simulink model "VDCHyd2022a"  (R2022a)
settings: Solver=daessc  StartTime=0.0  StopTime=simulationEndTime  FixedStep=0.001  RelTol=1e-2
values from neighbouring files (symbols this model uses):
  aux = thetaXrLB(i)    [initInertiaUpdate.m]
  Bc1_V = [0;0;0;0;0;0]    [InitializeSimulationParameters.m]
  Bc1_Vr = [0;0;0;0;0;0]    [InitializeSimulationParameters.m]
  D22Fr = [0;0;0;0;0;0]    [InitializeSimulationParameters.m]
  filtDF = init2ndOrderLowPassFilter(filtDF.cutOffFrequency,1,controller.dT)    [initializeLowPassFilters.m]
  filtDV = init2ndOrderLowPassFilter(filtDV.cutOffFrequency,1,controller.dT)    [initializeLowPassFilters.m]
  filtEnc = init2ndOrderLowPassFilter(filtEnc.cutOffFrequency,1,controller.dT)    [initializeLowPassFilters.m]
  filtPres = init2ndOrderLowPassFilter(filtPres.cutOffFrequency,1,controller.dT)    [initializeLowPassFilters.m]
  MODE = 1    [RUN_ME.m]
  s = tf('s')    [init2ndOrderLowPassFilter.m]
undefined symbols (not defined in the file or in its folder): B11_r_B11Tc1, B11_V, B11_Vr, B11Ftot_r, B12_r_B12Tc2, B12_Rot_Tc2, B12_U_Tc2, B12_V, B12_Vr, B12Ftot_r, B31_r_B31B41, B31_V, B31_Vr, B31FTot_r, B32_r_B32B42, B32_Rot_B42, B32_U_B42, B32_V, B32_Vr, B32FTot_r, B41_r_B41Tc1, B41_V, B41_Vr, B41FTot_r, B42_r_B42Tc2, B42_Rot_Tc2, B42_U_Tc2, B42_V, B42_Vr, B42FTot_r, B52_r_B52P32, B52_Rot_P32, B52_U_P32, B52_V, B52_Vr, B52Ftot_r, Bc1_r_Bc1B11, Bc1_r_Bc1B31, Bc1FTot_r, Bc2_r_Bc2B12, Bc2_r_Bc2B32, Bc2_Rot_B12, Bc2_Rot_B32, Bc2_U_B12, Bc2_U_B32, Bc2_V, Bc2_Vr, Bc2Tot_r, controller, cyl1, cyl2, cylT2, D22_V, D22_Vr, DiscIntNeverNeededParam, dq1, dq11, dq11r, dq12, dq12r ... (+119)
libraries: sm_lib x34, nesl_utility x15, simulink x11, dspinverses x1
(part 1 of 12)
settings Model: SimulationMode=accelerator  Creator=liikaneh  LastModifiedBy=pvgope
settings SolverCC: AlgebraicLoopSolver=TrustRegion
settings OptimizationCC: DefaultParameterBehavior=Inlined  GainParamInheritBuiltInType=on  UseFloatMulNetSlope=on  InlineInvariantSignals=on  EfficientFloat2IntCast=on
settings DebuggingCC: ReadBeforeWriteMsg=DisableAll  WriteAfterWriteMsg=DisableAll  WriteAfterReadMsg=DisableAll  MultiTaskDSMMsg=none  UnconnectedInputMsg=warning  UnconnectedOutputMsg=warning  UnconnectedLineMsg=warning  SFMachineParentedDataDiag=warning  ArithmeticOperatorsInVariantConditions=warning
settings ModelReferenceCC: UpdateModelReferenceTargets=IfOutOfDate
settings SFSimCC: SFSimEcho=off  SimUseLocalCustomCode=off  CustomCodeUndefinedFunction=UseInterfaceOnly
settings RTWCC: RTWUseLocalCustomCode=off  BuildConfiguration=Faster Runs  DLArmComputeVersion=19.05
settings GRTTargetCC: MatFileLogging=off  SupportNonFinite=off
settings DiagnosticsConfigSet: SimMechanicsRigidlyBoundBlock=none

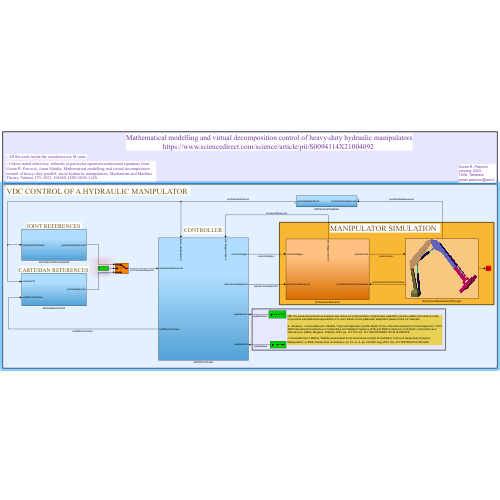
[thumbnail: Simulink's stored preview of the top-level diagram]
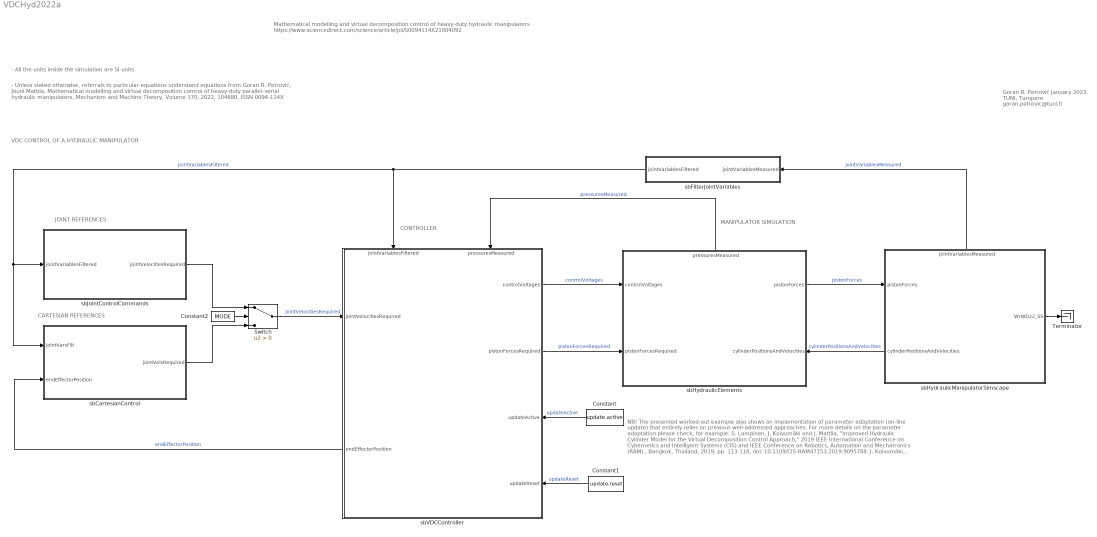
== system VDCHyd2022a ==
  note: NB! The presented worked-out example also shows an implementation of parameter adaptation (on-line update) that entirely relies on previous well-addressed approaches. For more details on the parameter adaptation please check, for example:
      |
      | S. Lampinen, J. Koivumäki and J. Mattila, "Improved Hydraulic Cylinder Model for the Virtual Decomposition Control Approach," 2019 IEEE International Conference on Cybernetics and Intelligent Systems (CIS) and IEEE Conference on Robotics, Automation and Mechatronics (RAM) , Bangkok, Thailand, 2019, pp. 113-118, doi: 10.1109/CIS-RAM47153.2019.9095788.
      |
      | J. Koivumäki and J. Mattila, "Stability-Guaranteed Force-Sensorless Contact Force/Motion Control of Heavy-Duty Hydraulic Manipulators," in IEEE Transactions on Robotics , vol. 31, no. 4, pp. 918-935, Aug. 2015, doi: 10.1109/TRO.2015.2441492.
  note: Mathematical modelling and virtual decomposition control of heavy-duty hydraulic manipulators
      | https://www.sciencedirect.com/science/article/pii/S0094114X21004092
  note: Goran R. Petrović
      | January 2023.
      | TUNI, Tampere
      | goran.petrovic@tuni.fi
  note: - All the units inside the simulation are SI units.
  note: - Unless stated otherwise, referrals to particular equations understand equations from Goran R. Petrović, Jouni Mattila, Mathematical modelling and virtual decomposition control of heavy-duty parallel–serial hydraulic manipulators, Mechanism and Machine Theory, Volume 170, 2022, 104680, ISSN 0094-114X
  note: MANIPULATOR SIMULATION
  note: VDC CONTROL OF A HYDRAULIC MANIPULATOR
  note: JOINT REFERENCES
  note: CARTESIAN REFERENCES
  note: CONTROLLER
  Constant : Constant  Value=update.active
  Constant1 : Constant  Value=update.reset
  Constant2 : Constant  Value=MODE
  Switch : Switch  Criteria=u2 > Threshold  SaturateOnIntegerOverflow=off  InputSameDT=off
  Terminator : Terminator
  sbCartesianControl : Subsystem
  sbFilterJointVariables : Subsystem
  sbHydraulicElements : Subsystem
      settings: PortSchema="{\"entries\":[{\"content\":{\"sides\":[{\"content\":{\"connectorIds\":[\"In1\",\"In2\"]},\"type\":\"ConnectorPlacement.EquallySpacedRectSide\",\"uuid\":\"d7e88d44-ea3b-4e6f-b434-d63e26d49c99\"},{\"content\":{\"connectorIds\":[\"Out1\",\"In3\"],\"side\":\"RIGHT\"},\"type\":\"ConnectorPlacement.EquallySpacedRectSide\",\"uuid\":\"625eb6db-a413-4233-8471-3960265b5680\"},{\"content\":{\"connectorIds\":[\"Out2\"],\"side\":\"TOP\"},\"type\":\"ConnectorPlacement.EquallySpacedRectSide\",\"uuid\":\"1363109f-1b18-4a4e-ba16-4e74caafe6c6\"}]},\"type\":\"ConnectorPlacement.EquallySpacedConnector\",\"uuid\":\"f039fec2-5503-4fd9-bf11-cf75dff43144\"}],\"packageUris\":[\"http://schema.mathworks.com/mf0/Connector/R2020b\"],\"version\":\"1.0\"}"
  sbHydraulicManipulatorSimscape : Subsystem
      settings: PortSchema="{\"entries\":[{\"content\":{\"sides\":[{\"content\":{\"connectorIds\":[\"In1\",\"Out3\"]},\"type\":\"ConnectorPlacement.EquallySpacedRectSide\",\"uuid\":\"f7b00952-2d51-484f-abea-a7edf7f1803a\"},{\"content\":{\"connectorIds\":[\"Out1\"],\"side\":\"RIGHT\"},\"type\":\"ConnectorPlacement.EquallySpacedRectSide\",\"uuid\":\"cec57a8d-f407-43fc-b54f-695abbd67ebc\"},{\"content\":{\"connectorIds\":[\"Out2\"],\"side\":\"TOP\"},\"type\":\"ConnectorPlacement.EquallySpacedRectSide\",\"uuid\":\"36c8b0b2-f27a-4d8c-8e2c-18a80d711d3e\"}]},\"type\":\"ConnectorPlacement.EquallySpacedConnector\",\"uuid\":\"9ce8286e-5e91-4ec7-b364-968722180a48\"}],\"packageUris\":[\"http://schema.mathworks.com/mf0/Connector/R2020b\"],\"version\":\"1.0\"}"
      mask Display: image('$imagefile'); % Use "Edit Image" on toolstrip to change.
  sbJointControlCommands : Subsystem
  sbVDCController : Subsystem
      settings: PortSchema="{\"entries\":[{\"content\":{\"sides\":[{\"content\":{\"connectorIds\":[\"In1\",\"Out3\"]},\"type\":\"ConnectorPlacement.EquallySpacedRectSide\",\"uuid\":\"7b05da7d-8e98-4260-b965-883aeff80f6d\"},{\"content\":{\"connectorIds\":[\"Out1\",\"Out2\",\"In4\",\"In5\"],\"side\":\"RIGHT\"},\"type\":\"ConnectorPlacement.EquallySpacedRectSide\",\"uuid\":\"bab503f6-0cf2-4d25-8612-166524dadf44\"},{\"content\":{\"connectorIds\":[\"In2\",\"In3\"],\"side\":\"TOP\"},\"type\":\"ConnectorPlacement.EquallySpacedRectSide\",\"uuid\":\"dc9bf139-dfcc-4316-b9ab-c299ea19db13\"}]},\"type\":\"ConnectorPlacement.EquallySpacedConnector\",\"uuid\":\"a723f5e0-c36b-4f3a-b452-df4ada5825ab\"}],\"packageUris\":[\"http://schema.mathworks.com/mf0/Connector/R2020b\"],\"version\":\"1.0\"}"
  wires:
  sbVDCController/1(controlVoltages) -> sbHydraulicElements/1(controlVoltages)  "controlVoltages"
  sbHydraulicElements/1(pistonForces) -> sbHydraulicManipulatorSimscape/1(pistonForces)  "pistonForces"
  Switch/1 -> sbVDCController/1(jointVelocitiesRequired)  "jointVelocitiesRequired"
  sbHydraulicManipulatorSimscape/2(jointVariablesMeasured) -> sbFilterJointVariables/1(jointVariablesMeasured)  "jointVariablesMeasured"
  sbFilterJointVariables/1(jointVariablesFiltered) -> sbVDCController/2(jointVariablesFiltered), sbCartesianControl/1(jointVarsFilt), sbJointControlCommands/1(jointVariablesFiltered)  "jointVariablesFiltered"
  sbHydraulicManipulatorSimscape/1(WrWD22_SS) -> Terminator/1
  sbVDCController/2(pistonForcesRequired) -> sbHydraulicElements/2(pistonForcesRequired)  "pistonForcesRequired"
  sbHydraulicElements/2(pressuresMeasured) -> sbVDCController/3(pressuresMeasured)  "pressuresMeasured"
  Constant/1 -> sbVDCController/4(updateActive)  "updateActive"
  Constant1/1 -> sbVDCController/5(updateReset)  "updateReset"
  sbVDCController/3(endEffectorPosition) -> sbCartesianControl/2(endEffectorPosition)  "endEffectorPosition"
  sbHydraulicManipulatorSimscape/3(cylinderPositionsAndVelocities) -> sbHydraulicElements/3(cylinderPositionsAndVelocities)  "cylinderPositionsAndVelocities"
  sbJointControlCommands/1(jointVelocitiesRequired) -> Switch/1
  sbCartesianControl/1(jointVelsRequired) -> Switch/3
  Constant2/1 -> Switch/2

== system VDCHyd2022a/sbCartesianControl ==
  note: Pass to outputs...
  note: Process data...
  note: Select from existing buses...
  note: X^{'}_r = X^{'}_d + \lambda_X (X - X_d)
  note: (3.22) W. H. Zhu, Virtual decomposition control: toward hyper degrees of freedom robots, pp. 51
  note: (3.21) W. H. Zhu, Virtual decomposition control: toward hyper degrees of freedom robots, pp. 51
  note: (3.21) W. H. Zhu, Virtual decomposition control: toward hyper degrees of freedom robots, pp. 51
  note: Get inputs...
  note: Y^{'}_r = Y^{'}_d + \lambda_Y (Y - Y_d)
  note: q^{'}_r = J^{ -1} V^{'}_r
  note: Compare desired and obtained TCP positions.
  jointVarsFilt : Inport
  endEffectorPosition : Inport  Port=2
  Bus Selector : BusSelector  OutputSignals=theta1Filtered,theta2Filtered,xt2Filtered
  Demux2 : Demux  Outputs=3
  From Workspace : FromWorkspace  VariableName=[pathPlanner.timeVector' pathPlanner.posDesCart(1,1:end)']  SampleTime=controller.dT
  From Workspace1 : FromWorkspace  VariableName=[pathPlanner.timeVector' pathPlanner.posDesCart(2,1:end)']  SampleTime=controller.dT
  From Workspace2 : FromWorkspace  VariableName=[pathPlanner.timeVector' pathPlanner.velDesCart(1,1:end)']  SampleTime=controller.dT
  From Workspace3 : FromWorkspace  VariableName=[pathPlanner.timeVector' pathPlanner.velDesCart(2,1:end)']  SampleTime=controller.dT
  Gain : Gain  Gain=controller.lamX
  Gain1 : Gain  Gain=controller.lamY
  Mux1 : Mux  Inputs=2
  Product : Product  Multiplication=Matrix(*)
  Pseudoinverse : dspinverses/Pseudoinverse  wanterr=off  SimulateUsing=Interpreted execution
      settings: SourceProductBaseCode=DS
  Scope : Scope  NumInputPorts=2
  Scope1 : Scope  NumInputPorts=2
  Sum3 : Sum  Inputs=|+-
  Sum4 : Sum  Inputs=|+-
  Sum5 : Sum  Inputs=|++
  Sum6 : Sum  Inputs=|++
  Terminator1 : Terminator
  velocityJacobianFunction : MATLAB Function  TreatAsAtomicUnit=on
  jointVelsRequired : Outport
  wires:
  [xt2Filt] -> velocityJacobianFunction/3(xt2)  "xt2Filt"
  [theta2Filt] -> velocityJacobianFunction/2(theta2)  "theta2Filt"
  Product/1 -> [jointVelsRequired]
  Mux1/1 -> Product/2
  velocityJacobianFunction/1(J) -> Pseudoinverse/1
  [theta1Filt] -> velocityJacobianFunction/1(theta1)  "theta1Filt"
  Pseudoinverse/1 -> Product/1
  [jointVelsRequired] -> jointVelsRequired/1  "jointVelsRequired"
  [XVelReq] -> Mux1/1
  [YVelReq] -> Mux1/2
  [XDes] -> Sum3/1
  [X] -> Sum3/2
  [YDes] -> Sum4/1
  [Y] -> Sum4/2
  Sum3/1 -> Gain/1
  Sum4/1 -> Gain1/1
  Gain/1 -> Sum5/1
  Gain1/1 -> Sum6/1
  [XVelDes] -> Sum5/2
  [YVelDes] -> Sum6/2
  Sum5/1 -> [XVelReq]
  Sum6/1 -> [YVelReq]
  [X] -> Scope/2
  [XDes] -> Scope/1
  [YDes] -> Scope1/1
  [Y] -> Scope1/2
  From Workspace/1 -> [XDes]
  From Workspace1/1 -> [YDes]
  From Workspace3/1 -> [YVelDes]
  From Workspace2/1 -> [XVelDes]
  [jointVarsFilt] -> Bus Selector/1  "jointVarsFilt"
  Bus Selector/3 -> [xt2Filt]  "<xt2Filtered>"
  Bus Selector/2 -> [theta2Filt]  "<theta2Filtered>"
  Bus Selector/1 -> [theta1Filt]  "<theta1Filtered>"
  Demux2/1 -> [X]  "X"
  Demux2/2 -> [Y]  "Y"
  Demux2/3 -> Terminator1/1
  [endEffectorPosition] -> Demux2/1  "WrWD22"
  jointVarsFilt/1 -> [jointVarsFilt]  "jointVarsFilt"
  endEffectorPosition/1 -> [endEffectorPosition]  "WrWD22"

== system VDCHyd2022a/sbFilterJointVariables ==
  jointVariablesMeasured : Inport  OutDataTypeStr=double  PortDimensions=3  SampleTime=controller.dT
  Bus Creator : BusCreator  Inputs=theta1Filtered,theta2Filtered,xt2Filtered
  Bus Selector : BusSelector  OutputSignals=theta1Measured,theta2Measured,xt2Measured
  sbTheta1LowPassFilter : Subsystem
  sbTheta2LowPassFilter : Subsystem
  sbxt2LowPassFilter : Subsystem
  jointVariablesFiltered : Outport  OutDataTypeStr=double  PortDimensions=3  SampleTime=controller.dT
  wires:
  sbxt2LowPassFilter/1(xt2Filtered) -> Bus Creator/3  "xt2Filtered"
  sbTheta2LowPassFilter/1(theta2Filtered) -> Bus Creator/2  "theta2Filtered"
  sbTheta1LowPassFilter/1(theta1Filtered) -> Bus Creator/1  "theta1Filtered"
  Bus Selector/2 -> sbTheta2LowPassFilter/1(theta2Measured)  "<theta2Measured>"
  Bus Selector/1 -> sbTheta1LowPassFilter/1(theta1Measured)  "<theta1Measured>"
  Bus Selector/3 -> sbxt2LowPassFilter/1(xt2Measured)  "<xt2Measured>"
  jointVariablesMeasured/1 -> Bus Selector/1  "jointVariablesMeasured"
  Bus Creator/1 -> jointVariablesFiltered/1  "jointVariablesFiltered"

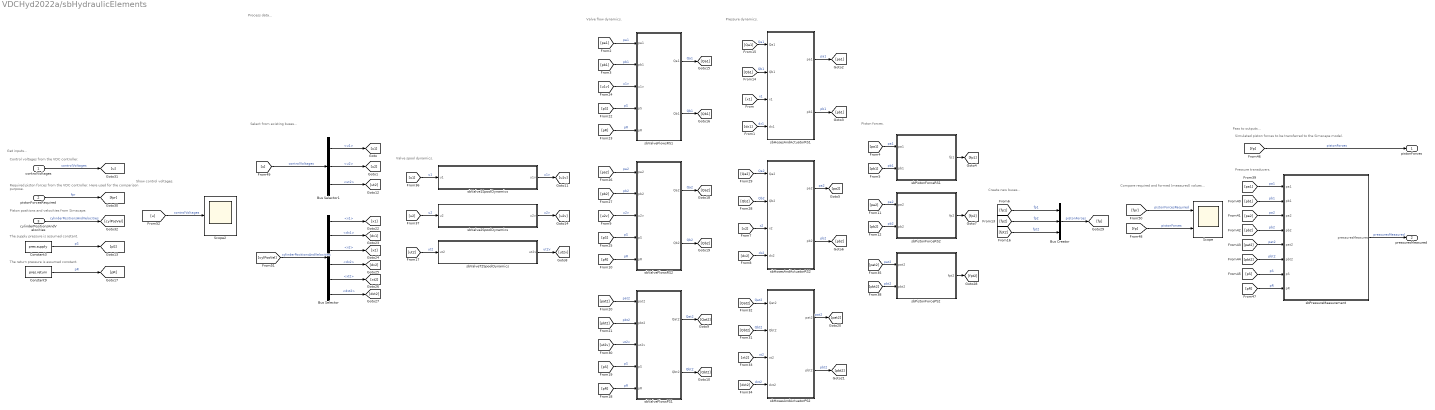
== system VDCHyd2022a/sbHydraulicElements ==
  note: Pass to outputs...
  note: Process data...
  note: Simulated piston forces to be transferred to the Simscape model.
  note: Pressure transducers.
  note: Create new buses...
  note: Select from existing buses...
  note: Piston positions and velocities from Simscape.
  note: Control voltages from the VDC controller.
  note: Required piston forces from the VDC controller.
      | Here used for the comparison purpose.
  note: Get inputs...
  note: The supply pressure is assumed constant.
  note: Valve spool dynamics.
  note: The return pressure is assumed constant.
  note: Piston forces.
  note: Pressure dynamics.
  note: Valve flow dynamics.
  note: Compare required and formed (measured) values...
  note: Show control voltages.
  controlVoltages : Inport
  pistonForcesRequired : Inport  Port=2
  cylinderPositionsAndVelocities : Inport  Port=3
  Bus Creator : BusCreator  Inputs=fp1,fp2,fpt2
  Bus Selector : BusSelector  OutputSignals=x1,dx1,x2,dx2,xt2,dxt2
  Bus Selector1 : BusSelector  OutputSignals=u1,u2,ut2
  Constant3 : Constant  Value=pres.supply
  Constant9 : Constant  Value=pres.return
  Scope : Scope  NumInputPorts=2
  Scope2 : Scope
  sbHosesAndActuatorPS2 : Subsystem
  sbHosesAndActuatorRS1 : Subsystem
  sbHosesAndActuatorRS2 : Subsystem
  sbPistonForcePS2 : Subsystem
  sbPistonForceRS1 : Subsystem
  sbPistonForceRS2 : Subsystem
  sbPressureMeasurement : Subsystem
  sbValve1SpoolDynamics : Subsystem
  sbValve2SpoolDynamics : Subsystem
  sbValveFlowsPS1 : Subsystem
  sbValveFlowsRS1 : Subsystem
  sbValveFlowsRS2 : Subsystem
  sbValveT2SpoolDynamics : Subsystem
  pistonForces : Outport
  pressuresMeasured : Outport  Port=2
  wires:
  [u1v] -> sbValveFlowsRS1/3(u1v)  "u1v"
  [Qb2] -> sbHosesAndActuatorRS2/2(Qb2)  "Qb2"
  sbValveFlowsRS2/1(Qa2) -> [Qa2]  "Qa2"
  [u2] -> sbValve2SpoolDynamics/1(u2)  "u2"
  [pS] -> sbValveFlowsRS1/4(pS)  "pS"
  [u2v] -> sbValveFlowsRS2/3(u2v)  "u2v"
  sbValveFlowsRS2/2(Qb2) -> [Qb2]  "Qb2"
  [dx2] -> sbHosesAndActuatorRS2/4(dx2)  "dx2"
  [pa2] -> sbValveFlowsRS2/1(pa2)  "pa2"
  [pb1] -> sbValveFlowsRS1/2(pb1)  "pb1"
  [dx1] -> sbHosesAndActuatorRS1/4(dx1)  "dx1"
  sbValveFlowsRS1/1(Qa1) -> [Qa1]  "Qa1"
  [pa1] -> sbValveFlowsRS1/1(pa1)  "pa1"
  [pR] -> sbValveFlowsRS1/5(pR)  "pR"
  sbHosesAndActuatorRS2/2(pb2) -> [pb2]  "pb2"
  [Qa2] -> sbHosesAndActuatorRS2/1(Qa2)  "Qa2"
  [Qa1] -> sbHosesAndActuatorRS1/1(Qa1)  "Qa1"
  Constant9/1 -> [pR]  "pR"
  [Qb1] -> sbHosesAndActuatorRS1/2(Qb1)  "Qb1"
  [pb2] -> sbValveFlowsRS2/2(pb2)  "pb2"
  sbHosesAndActuatorRS1/1(pa1) -> [pa1]  "pa1"
  [x2] -> sbHosesAndActuatorRS2/3(x2)  "x2"
  sbValve1SpoolDynamics/1(u1v) -> [u1v]  "u1v"
  [x1] -> sbHosesAndActuatorRS1/3(x1)  "x1"
  [u1] -> sbValve1SpoolDynamics/1(u1)  "u1"
  sbHosesAndActuatorRS1/2(pb1) -> [pb1]  "pb1"
  Constant3/1 -> [pS]  "pS"
  [pR] -> sbValveFlowsRS2/5(pR)  "pR"
  sbValve2SpoolDynamics/1(u2v) -> [u2v]  "u2v"
  [pS] -> sbValveFlowsRS2/4(pS)  "pS"
  sbValveFlowsRS1/2(Qb1) -> [Qb1]  "Qb1"
  sbHosesAndActuatorRS2/1(pa2) -> [pa2]  "pa2"
  [fp1] -> Bus Creator/1  "fp1"
  [fp2] -> Bus Creator/2  "fp2"
  [fpt2] -> Bus Creator/3  "fpt2"
  sbValveT2SpoolDynamics/1(ut2v) -> [ut2v]  "ut2v"
  [ut2] -> sbValveT2SpoolDynamics/1(ut2)  "ut2"
  [pat2] -> sbValveFlowsPS1/1(pat2)  "pat2"
  [ut2v] -> sbValveFlowsPS1/3(ut2v)  "ut2v"
  sbValveFlowsPS1/2(Qbt2) -> [Qbt2]  "Qbt2"
  [pR] -> sbValveFlowsPS1/5(pR)  "pR"
  [pS] -> sbValveFlowsPS1/4(pS)  "pS"
  sbValveFlowsPS1/1(Qat2) -> [Qat2]  "Qat2"
  [pbt2] -> sbValveFlowsPS1/2(pbt2)  "pbt2"
  sbHosesAndActuatorPS2/1(pat2) -> [pat2]  "pat2"
  [xt2] -> sbHosesAndActuatorPS2/3(xt2)  "xt2"
  [Qat2] -> sbHosesAndActuatorPS2/1(Qat2)  "Qat2"
  sbHosesAndActuatorPS2/2(pbt2) -> [pbt2]  "pbt2"
  [dxt2] -> sbHosesAndActuatorPS2/4(dxt2)  "dxt2"
  [Qbt2] -> sbHosesAndActuatorPS2/2(Qbt2)  "Qbt2"
  Bus Creator/1 -> [fp]  "pistonForces"
  [fp] -> pistonForces/1  "pistonForces"
  [fpr] -> Scope/1  "pistonForcesRequired"
  [fp] -> Scope/2  "pistonForces"
  pistonForcesRequired/1 -> [fpr]  "fpr"
  Bus Selector1/2 -> [u2]  "<u2>"
  Bus Selector1/1 -> [u1]  "<u1>"
  [u] -> Bus Selector1/1  "controlVoltages"
  Bus Selector1/3 -> [ut2]  "<ut2>"
  controlVoltages/1 -> [u]  "controlVoltages"
  Bus Selector/6 -> [dxt2]  "<dxt2>"
  Bus Selector/4 -> [dx2]  "<dx2>"
  Bus Selector/2 -> [dx1]  "<dx1>"
  Bus Selector/1 -> [x1]  "<x1>"
  Bus Selector/5 -> [xt2]  "<xt2>"
  Bus Selector/3 -> [x2]  "<x2>"
  [cylPosVel] -> Bus Selector/1  "cylinderPositionsAndVelocities"
  cylinderPositionsAndVelocities/1 -> [cylPosVel]  "cylinderPositionsAndVelocities"
  [u] -> Scope2/1  "controlVoltages"
  [pa1] -> sbPistonForceRS1/1(pa1)  "pa1"
  [pb1] -> sbPistonForceRS1/2(pb1)  "pb1"
  sbPistonForceRS1/1(fp1) -> [fp1]
  [pa1] -> sbPressureMeasurement/1(pa1)  "pa1"
  [pb1] -> sbPressureMeasurement/2(pb1)  "pb1"
  [pa2] -> sbPressureMeasurement/3(pa2)  "pa2"
  [pb2] -> sbPressureMeasurement/4(pb2)  "pb2"
  [pat2] -> sbPressureMeasurement/5(pat2)  "pat2"
  [pbt2] -> sbPressureMeasurement/6(pbt2)  "pbt2"
  [pS] -> sbPressureMeasurement/7(pS)  "pS"
  [pR] -> sbPressureMeasurement/8(pR)  "pR"
  sbPressureMeasurement/1(pressuresMeasured) -> pressuresMeasured/1  "pressuresMeasured"
  [pat2] -> sbPistonForcePS2/1(pat2)  "pat2"
  [pbt2] -> sbPistonForcePS2/2(pbt2)  "pbt2"
  sbPistonForcePS2/1(fpt2) -> [fpt2]
  [pa2] -> sbPistonForceRS2/1(pa2)  "pa2"
  [pb2] -> sbPistonForceRS2/2(pb2)  "pb2"
  sbPistonForceRS2/1(fp2) -> [fp2]

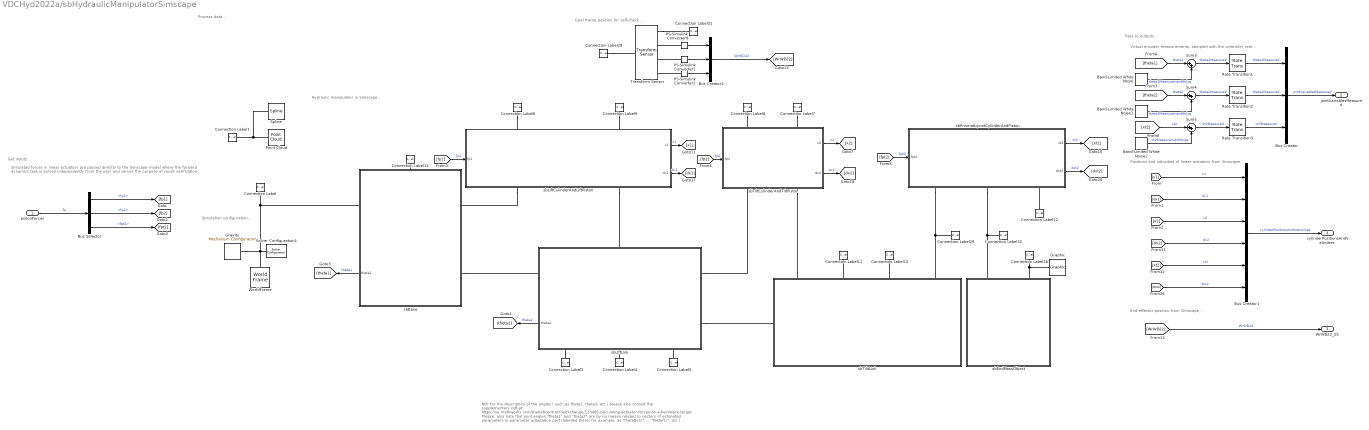
== system VDCHyd2022a/sbHydraulicManipulatorSimscape ==
  note: NB! For the description of the angles ( such as theta1, theta2, etc.) please also consult the supplementary pdf at:
      | https://se.mathworks.com/matlabcentral/fileexchange/123465-calculating-actuator-forces-on-a-hardware-target.
      | Please, also note that joint angles "theta1" and "theta2" are by no means related to vectors of estimated parameters in parameter adaptation part (labelled there, for example, as "thetaBc1r",... "thetaf1r", etc.)
  note: Get inputs...
  note: Process data...
  note: Simulated forces in linear actuators are passed directly to the Simscape model
      | where the forward dynamics task is solved independently from the user and
      | serves the purpose of result verification.
  note: Hydraulic manipulator in Simscape...
  note: Simulation configuration...
  note: Pass to outputs...
  note: Virtual encoder measurements, sampled with the controller rate...
  note: Positions and velocities of linear actuators from Simscape...
  note: End-effector position from Simscape...
  note: Goal frame position for self-check...
  pistonForces : Inport
  Band-Limited White Noise : simulink/Sources/Band-Limited White Noise  Cov=encoder.measNoisePower  Ts=controller.dT  seed=[23341]
  Band-Limited White Noise1 : simulink/Sources/Band-Limited White Noise  Cov=encoder.measNoisePower  Ts=controller.dT  seed=[23341]
  Band-Limited White Noise2 : simulink/Sources/Band-Limited White Noise  Cov=encoder.measNoisePower  Ts=controller.dT  seed=[23341]
  Bus Creator : BusCreator  Inputs=theta1Measured,theta2Measured,xt2Measured
  Bus Creator1 : BusCreator  Inputs=x1,dx1,x2,dx2,xt2,dxt2
  Bus Creator2 : BusCreator  Inputs=3
  Bus Selector : BusSelector  OutputSignals=fp1,fp2,fpt2
  Connection Label : ConnectionLabel  Label=W
  Connection Label1 : ConnectionLabel  Label=W
  Connection Label11 : ConnectionLabel  Label=B12
  Connection Label12 : ConnectionLabel  Label=B52
  Connection Label14 : ConnectionLabel  Label=Bc1
  Connection Label15 : ConnectionLabel  Label=Tc2
  Connection Label16 : ConnectionLabel  Label=D22
  Connection Label28 : ConnectionLabel  Label=W
  Connection Label29 : ConnectionLabel  Label=P22
  Connection Label3 : ConnectionLabel  Label=Tc1
  Connection Label31 : ConnectionLabel  Label=D22
  Connection Label32 : ConnectionLabel  Label=P32
  Connection Label4 : ConnectionLabel  Label=B11
  Connection Label5 : ConnectionLabel  Label=Bc2
  Connection Label6 : ConnectionLabel  Label=B31
  Connection Label7 : ConnectionLabel  Label=B42
  Connection Label8 : ConnectionLabel  Label=B32
  Connection Label9 : ConnectionLabel  Label=B41
  Graphic : sm_lib/Body Elements/Graphic  GraphicType=Marker  MarkerShape=Frame  MarkerSize=50  GraphicVisPropType=SimpleVisualProperties  GraphicDiffuseColor=[0.9294 0.6941 0.1255]  GraphicSpecularColor=[0.5 0.5 0.5 1.0]  GraphicAmbientColor=[0.15 0.15 0.15 1.0]  GraphicEmissiveColor=[0.0 0.0 0.0 1.0]  GraphicShininess=75  GraphicOpacity=1.0
  Gravity : sm_lib/Utilities/Mechanism Configuration  UniformGravity=Constant  GravityVector=-gravity.Wg  GravityUnits=m/s^2  LinearizationDelta=0.001  JointModeTransitionNonlinearIterations=2
  PS-Simulink Converter1 : nesl_utility/PS-Simulink Converter  PhysicalDomain=network_engine_domain  SubClassName=ps_output  LeftPortType=input  RightPortType=output  PseudoPeriodic=off  Frequencies=[]  VectorFormat=1-D array  Unit=inherit  AffineConversion=off
      settings: SourceProductBaseCode=SS,PW,VE
  PS-Simulink Converter2 : nesl_utility/PS-Simulink Converter  PhysicalDomain=network_engine_domain  SubClassName=ps_output  LeftPortType=input  RightPortType=output  PseudoPeriodic=off  Frequencies=[]  VectorFormat=1-D array  Unit=inherit  AffineConversion=off
      settings: SourceProductBaseCode=SS,PW,VE
  PS-Simulink Converter8 : nesl_utility/PS-Simulink Converter  PhysicalDomain=network_engine_domain  SubClassName=ps_output  LeftPortType=input  RightPortType=output  PseudoPeriodic=off  Frequencies=[]  VectorFormat=1-D array  Unit=inherit  AffineConversion=off
      settings: SourceProductBaseCode=SS,PW,VE
  Point Cloud : sm_lib/Curves and Surfaces/Point Cloud  CoordinatesMatrix=pointCloudMatrix  CoordinatesMatrixUnits=m  GraphicType=MarkerCloud  GraphicSphereRadius=2e-2  GraphicSphereRadiusUnits=m  GraphicVisPropType=SimpleVisualProperties  GraphicDiffuseColor=[1 1 0.06667]  GraphicOpacity=1.0  GraphicSpecularColor=[0.5 0.5 0.5 1.0]  GraphicAmbientColor=[0.15 0.15 0.15 1.0]  GraphicEmissiveColor=[0.0 0.0 0.0 1.0]  GraphicShininess=75
      settings: SourceProductBaseCode=MS
  Rate Transition1 : RateTransition  InitialCondition=initVals.theta10  OutPortSampleTime=controller.dT
  Rate Transition2 : RateTransition  InitialCondition=initVals.theta20  OutPortSampleTime=controller.dT
  Rate Transition3 : RateTransition  InitialCondition=initVals.xt20  OutPortSampleTime=controller.dT
  Solver Configuration1 : nesl_utility/Solver Configuration  PhysicalDomain=network_engine_domain  SubClassName=solver  LeftPortType=input  RightPortType=generic  Tones=[]  Harmonics=[]  SimulateNoise=off  Profile=off  UseLocalSampling=off  EnableSwitchedLinearOptims=on  FrequencyDomain=off  UseCCode=off  RelTol=0.001  AbsTol=1e-06  MinStep=1e-09  ToWorkspace=off  RevertToSquareIcSolve=off  NumHomotopyIterations=100  PhasorMode=off  PhasorModeNumHarmonics=1  IndexReductionMethod=DerivativeReplacement  DoDC=on  ResidualTolerance=1e-9  UseLocalSolver=off  LocalSolverChoice=NE_TRAPEZOIDAL_ADVANCER  LocalSolverSampleTime=0.002  DoFixedCost=off  MaxNonlinIter=3  MaxModeIter=2  ComputeImpulses=off  ImpulseIterations=2  LinearAlgebra=Sparse  LinearAlgebraNumThread=0  EquationFormulation=NE_TIME_EF  DelaysMemoryBudget=1024  AutomaticFiltering=on  FilteringTimeConstant=0.001  PartitionStorageMethod=AS_NEEDED  PartitionMemoryBudget=1024  PartitionMethod=FAST
      settings: SourceProductBaseCode=SS,PW,VE
  Spline : sm_lib/Curves and Surfaces/Spline  GraphicAmbientColor=[0.15 0.15 0.15 1.0]  GraphicDiffuseColor=[0.0 0.0 0.0]  DataPoints=pointCloudMatrix  DataPointsUnits=m  GraphicEmissiveColor=[0.0 0.0 0.0 1.0]  EndConditionType=Natural  MarkerShape=Sphere  MarkerSize=10  GraphicType=FromGeometry  GraphicOpacity=1.0  GraphicShininess=75  GraphicSpecularColor=[0.5 0.5 0.5 1.0]  GraphicVisPropType=SimpleVisualProperties
  Sum3 : Sum  Inputs=|++
  Sum4 : Sum  Inputs=|++
  Sum5 : Sum  Inputs=|++
  Transform Sensor : sm_lib/Frames and Transforms/Transform Sensor  MeasurementFrame=NonRotatingBase  SenseAngle=off  SenseAxis=off  SenseAngle1=off  SenseAngle2=off  SenseAngle3=off  SenseQ=off  SenseR=off  SenseOmegaX=off  SenseOmegaY=off  SenseOmegaZ=off  SenseOmega1=off  SenseOmega2=off  SenseOmega3=off  SenseQDot=off  SenseRDot=off  SenseAlphaX=off  SenseAlphaY=off  SenseAlphaZ=off  SenseAlpha1=off  SenseAlpha2=off  SenseAlpha3=off  SenseQDDot=off  SenseRDDot=off  SenseX=on  SenseY=on  SenseZ=on  SenseRad=off  SenseAzim=off  SenseDist=off  SenseInc=off  SenseXDot=off  SenseYDot=off  SenseZDot=off  SenseRadDot=off  SenseAzimDot=off  SenseDistDot=off  SenseIncDot=off  SenseXDDot=off  SenseYDDot=off  SenseZDDot=off  SenseRadDDot=off  SenseAzimDDot=off  SenseDistDDot=off  SenseIncDDot=off
  WorldFrame : sm_lib/Frames and Transforms/World Frame
  sbBase : Subsystem
      settings: PortSchema="{\"entries\":[{\"content\":{\"sides\":[{\"content\":{\"connectorIds\":[\"LConn1\",\"Out1\"]},\"type\":\"ConnectorPlacement.EquallySpacedRectSide\",\"uuid\":\"74e7f3c6-cbce-4102-a556-47a2132f5eea\"},{\"content\":{\"connectorIds\":[\"RConn1\",\"RConn2\"],\"side\":\"RIGHT\"},\"type\":\"ConnectorPlacement.EquallySpacedRectSide\",\"uuid\":\"9dc74751-c8ff-4cb6-874a-dcd58e00de96\"},{\"content\":{\"connectorIds\":[\"LConn2\"],\"side\":\"TOP\"},\"type\":\"ConnectorPlacement.EquallySpacedRectSide\",\"uuid\":\"06e145de-a8a9-4531-940d-434d89c78f5b\"}]},\"type\":\"ConnectorPlacement.EquallySpacedConnector\",\"uuid\":\"f796a1f4-9531-411f-8f55-fdef488b8a52\"}],\"packageUris\":[\"http://schema.mathworks.com/mf0/Connector/R2020b\"],\"version\":\"1.0\"}"
  sbEndMassObject : Subsystem
      settings: PortSchema="{\"entries\":[{\"content\":{\"sides\":[{\"content\":{\"connectorIds\":[]},\"type\":\"ConnectorPlacement.EquallySpacedRectSide\",\"uuid\":\"c1652833-a888-40a4-a60e-17be9708feae\"},{\"content\":{\"connectorIds\":[],\"side\":\"RIGHT\"},\"type\":\"ConnectorPlacement.EquallySpacedRectSide\",\"uuid\":\"55671429-adc4-418e-b6f5-c624f049c776\"},{\"content\":{\"connectorIds\":[\"LConn1\",\"LConn2\"],\"side\":\"TOP\"},\"type\":\"ConnectorPlacement.EquallySpacedRectSide\",\"uuid\":\"549e793d-1b28-4f93-9706-f4524b8bc4e2\"}]},\"type\":\"ConnectorPlacement.EquallySpacedConnector\",\"uuid\":\"9a6e434f-5824-411f-a3a4-9b8ec603a501\"}],\"packageUris\":[\"http://schema.mathworks.com/mf0/Connector/19700101\"],\"version\":\"1.0\"}"
  sbLiftCylinderAndLiftPiston : Subsystem
      settings: PortSchema="{\"entries\":[{\"content\":{\"sides\":[{\"content\":{\"connectorIds\":[\"In1\"]},\"type\":\"ConnectorPlacement.EquallySpacedRectSide\",\"uuid\":\"a609877c-275e-4024-96c6-67831631fbf9\"},{\"content\":{\"connectorIds\":[\"Out1\",\"Out2\"],\"side\":\"RIGHT\"},\"type\":\"ConnectorPlacement.EquallySpacedRectSide\",\"uuid\":\"b747ace3-04d7-42f4-87a7-c62fd6093e0d\"},{\"content\":{\"connectorIds\":[\"LConn1\",\"LConn2\"],\"side\":\"TOP\"},\"type\":\"ConnectorPlacement.EquallySpacedRectSide\",\"uuid\":\"5f9db8d6-814e-4333-b197-0e9dcf847d3e\"},{\"content\":{\"connectorIds\":[\"RConn1\",\"RConn2\"],\"side\":\"BOTTOM\"},\"type\":\"ConnectorPlacement.EquallySpacedRectSide\",\"uuid\":\"d1d564c3-4146-4330-9936-8dd25e0cb4bf\"}]},\"type\":\"ConnectorPlacement.EquallySpacedConnector\",\"uuid\":\"d00f43c3-717c-4aa5-b919-dd57ad6708f7\"}],\"packageUris\":[\"http://schema.mathworks.com/mf0/Connector/R2020b\"],\"version\":\"1.0\"}"
  sbLiftLink : Subsystem
      settings: PortSchema="{\"entries\":[{\"content\":{\"sides\":[{\"content\":{\"connectorIds\":[\"LConn1\",\"LConn2\"]},\"type\":\"ConnectorPlacement.EquallySpacedRectSide\",\"uuid\":\"50668ed3-3246-41c6-a320-c5b34ebd86b6\"},{\"content\":{\"connectorIds\":[\"RConn1\",\"Out1\"],\"side\":\"RIGHT\"},\"type\":\"ConnectorPlacement.EquallySpacedRectSide\",\"uuid\":\"d76ddc23-e4dc-4bdf-9e15-3eadac6cf1e2\"},{\"content\":{\"connectorIds\":[\"LConn3\"],\"side\":\"TOP\"},\"type\":\"ConnectorPlacement.EquallySpacedRectSide\",\"uuid\":\"5458eee7-805c-4d74-888c-3f811d80880c\"},{\"content\":{\"connectorIds\":[\"RConn2\",\"RConn3\",\"RConn4\"],\"side\":\"BOTTOM\"},\"type\":\"ConnectorPlacement.EquallySpacedRectSide\",\"uuid\":\"6f630415-b321-44c9-a6f9-9daa6b5086dd\"}]},\"type\":\"ConnectorPlacement.EquallySpacedConnector\",\"uuid\":\"adbb0eba-5908-47e0-8cde-3ca3a2901b66\"}],\"packageUris\":[\"http://schema.mathworks.com/mf0/Connector/R2020b\"],\"version\":\"1.0\"}"
  sbPrismaticJointCylinderAndPiston : Subsystem
      settings: PortSchema="{\"entries\":[{\"content\":{\"sides\":[{\"content\":{\"connectorIds\":[\"In1\"]},\"type\":\"ConnectorPlacement.EquallySpacedRectSide\",\"uuid\":\"002196eb-b81c-4ad4-9df1-33c4ef5d5c77\"},{\"content\":{\"connectorIds\":[\"Out1\",\"Out2\"],\"side\":\"RIGHT\"},\"type\":\"ConnectorPlacement.EquallySpacedRectSide\",\"uuid\":\"e0d61efe-ea5d-4756-bea5-1d107b09975a\"},{\"content\":{\"connectorIds\":[],\"side\":\"TOP\"},\"type\":\"ConnectorPlacement.EquallySpacedRectSide\",\"uuid\":\"1a952641-c922-4f91-9854-1cf1d6e715db\"},{\"content\":{\"connectorIds\":[\"RConn1\",\"RConn2\",\"RConn3\"],\"side\":\"BOTTOM\"},\"type\":\"ConnectorPlacement.EquallySpacedRectSide\",\"uuid\":\"13c3128f-85d9-4df5-9ae2-f45a9cb5a20e\"}]},\"type\":\"ConnectorPlacement.EquallySpacedConnector\",\"uuid\":\"7bd12321-8448-494e-b8ce-fe2f63fec7f7\"}],\"packageUris\":[\"http://schema.mathworks.com/mf0/Connector/R2020b\"],\"version\":\"1.0\"}"
  sbTilitLink : Subsystem
      settings: PortSchema="{\"entries\":[{\"content\":{\"sides\":[{\"content\":{\"connectorIds\":[]},\"type\":\"ConnectorPlacement.EquallySpacedRectSide\",\"uuid\":\"3124f0ed-3daa-4e61-aa81-877c0a0fd3a0\"},{\"content\":{\"connectorIds\":[\"RConn1\"],\"side\":\"RIGHT\"},\"type\":\"ConnectorPlacement.EquallySpacedRectSide\",\"uuid\":\"bc27bd78-7de5-476c-8b4b-17e2ed4c2476\"},{\"content\":{\"connectorIds\":[\"LConn1\",\"LConn2\",\"LConn3\",\"LConn4\"],\"side\":\"TOP\"},\"type\":\"ConnectorPlacement.EquallySpacedRectSide\",\"uuid\":\"46b542cf-bb62-4410-9418-b726c84ee3f9\"}]},\"type\":\"ConnectorPlacement.EquallySpacedConnector\",\"uuid\":\"3938a7f2-fa69-42c9-abcf-1c8c25e9b66f\"}],\"packageUris\":[\"http://schema.mathworks.com/mf0/Connector/19700101\"],\"version\":\"1.0\"}"
  sbTiltCylinderAndTiltPiston : Subsystem
      settings: PortSchema="{\"entries\":[{\"content\":{\"sides\":[{\"content\":{\"connectorIds\":[\"In1\"]},\"type\":\"ConnectorPlacement.EquallySpacedRectSide\",\"uuid\":\"a609877c-275e-4024-96c6-67831631fbf9\"},{\"content\":{\"connectorIds\":[\"Out1\",\"Out2\"],\"side\":\"RIGHT\"},\"type\":\"ConnectorPlacement.EquallySpacedRectSide\",\"uuid\":\"b747ace3-04d7-42f4-87a7-c62fd6093e0d\"},{\"content\":{\"connectorIds\":[\"LConn1\",\"LConn2\"],\"side\":\"TOP\"},\"type\":\"ConnectorPlacement.EquallySpacedRectSide\",\"uuid\":\"5f9db8d6-814e-4333-b197-0e9dcf847d3e\"},{\"content\":{\"connectorIds\":[\"RConn1\",\"RConn2\"],\"side\":\"BOTTOM\"},\"type\":\"ConnectorPlacement.EquallySpacedRectSide\",\"uuid\":\"d1d564c3-4146-4330-9936-8dd25e0cb4bf\"}]},\"type\":\"ConnectorPlacement.EquallySpacedConnector\",\"uuid\":\"d00f43c3-717c-4aa5-b919-dd57ad6708f7\"}],\"packageUris\":[\"http://schema.mathworks.com/mf0/Connector/R2020b\"],\"version\":\"1.0\"}"
  WrWD22_SS : Outport
  jointVariablesMeasured : Outport  Port=2
  cylinderPositionsAndVelocities : Outport  Port=3
  wires:
  sbLiftCylinderAndLiftPiston/1(x1) -> [x1]  "x1"
  sbTiltCylinderAndTiltPiston/1(x2) -> [x2]  "x2"
  [fpt2] -> sbPrismaticJointCylinderAndPiston/1(fpt2)  "fpt2"
  sbPrismaticJointCylinderAndPiston/1(xt2) -> [xt2]  "xt2"
  [WrWD22] -> WrWD22_SS/1  "WrWD22"
  PS-Simulink Converter2/1 -> Bus Creator2/3
  PS-Simulink Converter8/1 -> Bus Creator2/1
  PS-Simulink Converter1/1 -> Bus Creator2/2
  Bus Creator2/1 -> [WrWD22]  "WrWD22"
  [fp1] -> sbLiftCylinderAndLiftPiston/1(fp1)  "fp1"
  [fp2] -> sbTiltCylinderAndTiltPiston/1(fp2)  "fp2"
  sbLiftCylinderAndLiftPiston/2(dx1) -> [dx1]  "dx1"
  sbTiltCylinderAndTiltPiston/2(dx2) -> [dx2]  "dx2"
  sbPrismaticJointCylinderAndPiston/2(dxt2) -> [dxt2]  "dxt2"
  [dxt2] -> Bus Creator1/6  "dxt2"
  [xt2] -> Bus Creator1/5  "xt2"
  [dx2] -> Bus Creator1/4  "dx2"
  [x2] -> Bus Creator1/3  "x2"
  [dx1] -> Bus Creator1/2  "dx1"
  [x1] -> Bus Creator1/1  "x1"
  Bus Creator1/1 -> cylinderPositionsAndVelocities/1  "cylinderPositionsAndVelocities"
  sbLiftLink/1(theta2) -> [theta2]  "theta2"
  sbBase/1(theta1) -> [theta1]  "theta1"
  [theta1] -> Sum3/1  "theta1"
  Band-Limited White Noise/1 -> Sum3/2  "theta1MeasurementNoise"
  [theta2] -> Sum4/1  "theta2"
  Band-Limited White Noise1/1 -> Sum4/2  "theta2MeasurementNoise"
  [xt2] -> Sum5/1  "xt2"
  Band-Limited White Noise2/1 -> Sum5/2  "xt2MeasurementNoise"
  Bus Creator/1 -> jointVariablesMeasured/1  "jointVariablesMeasured"
  Sum4/1 -> Rate Transition2/1  "theta2Measured"
  Rate Transition1/1 -> Bus Creator/1  "theta1Measured"
  Rate Transition2/1 -> Bus Creator/2  "theta2Measured"
  Rate Transition3/1 -> Bus Creator/3  "xt2Measured"
  pistonForces/1 -> Bus Selector/1  "fp"
  Bus Selector/3 -> [fpt2]  "<fpt2>"
  Bus Selector/2 -> [fp2]  "<fp2>"
  Bus Selector/1 -> [fp1]  "<fp1>"
  Sum3/1 -> Rate Transition1/1  "theta1Measured"
  Sum5/1 -> Rate Transition3/1  "xt2Measured"
  connections:
  Gravity/RConn1 -- sbBase/LConn1 -- Connection Label/LConn1 -- WorldFrame/RConn1 -- Solver Configuration1/RConn1
  sbLiftLink/LConn1 -- sbTiltCylinderAndTiltPiston/RConn1
  sbLiftLink/LConn2 -- sbTilitLink/RConn1
  sbTiltCylinderAndTiltPiston/RConn2 -- sbTilitLink/LConn4
  sbLiftCylinderAndLiftPiston/RConn2 -- sbLiftLink/LConn3
  sbBase/RConn2 -- sbLiftLink/RConn1
  sbLiftCylinderAndLiftPiston/RConn1 -- sbBase/RConn1
  sbLiftLink/RConn4 -- Connection Label3/LConn1
  Connection Label4/LConn1 -- sbLiftLink/RConn3
  Connection Label5/LConn1 -- sbLiftLink/RConn2
  Connection Label6/LConn1 -- sbLiftCylinderAndLiftPiston/LConn1
  Connection Label9/LConn1 -- sbLiftCylinderAndLiftPiston/LConn2
  Connection Label7/LConn1 -- sbTiltCylinderAndTiltPiston/LConn2
  Connection Label8/LConn1 -- sbTiltCylinderAndTiltPiston/LConn1
  Connection Label11/LConn1 -- sbTilitLink/LConn3
  Connection Label15/LConn1 -- sbTilitLink/LConn2
  Connection Label16/LConn1 -- Graphic/RConn1 -- sbEndMassObject/LConn2
  Connection Label14/LConn1 -- sbBase/LConn2
  Connection Label12/LConn1 -- sbPrismaticJointCylinderAndPiston/RConn3
  sbPrismaticJointCylinderAndPiston/RConn1 -- Connection Label29/LConn1 -- sbTilitLink/LConn1
  sbPrismaticJointCylinderAndPiston/RConn2 -- sbEndMassObject/LConn1 -- Connection Label32/LConn1
  PS-Simulink Converter1/LConn1 -- Transform Sensor/RConn3
  PS-Simulink Converter8/LConn1 -- Transform Sensor/RConn2
  PS-Simulink Converter2/LConn1 -- Transform Sensor/RConn4
  Connection Label28/LConn1 -- Transform Sensor/LConn1
  Transform Sensor/RConn1 -- Connection Label31/LConn1
  Point Cloud/LConn1 -- Spline/LConn1 -- Connection Label1/LConn1

== system VDCHyd2022a/sbJointControlCommands ==
  note: Pass to outputs...
  note: Compare desired and measured values...
  note: Process data...
  note: Get inputs...
  note: q_j^{'}_r = q_j^{'}_d + \lambda_j (q_j - q_{jd})
  note: (36)
  jointVariablesFiltered : Inport
  Bus Creator : BusCreator  Inputs=theta1VelocityRequired,theta2VelocityRequired,xt2VelocityRequired
  Bus Selector : BusSelector  OutputSignals=theta1Filtered,theta2Filtered,xt2Filtered
  Discrete-Time Integrator : DiscreteIntegrator  InitialCondition=initVals.theta10  SampleTime=controller.dT  UpperSaturationLimit=1  LowerSaturationLimit=-1  ICPrevOutput=DiscIntNeverNeededParam  ICPrevScaledInput=DiscIntNeverNeededParam
  Discrete-Time Integrator1 : DiscreteIntegrator  InitialCondition=initVals.xt20  SampleTime=controller.dT  UpperSaturationLimit=1  LowerSaturationLimit=-1  ICPrevOutput=DiscIntNeverNeededParam  ICPrevScaledInput=DiscIntNeverNeededParam
  Discrete-Time Integrator3 : DiscreteIntegrator  InitialCondition=initVals.theta20  SampleTime=controller.dT  UpperSaturationLimit=1  LowerSaturationLimit=-1  ICPrevOutput=DiscIntNeverNeededParam  ICPrevScaledInput=DiscIntNeverNeededParam
  Gain : Gain  Gain=controller.lamTh1
  Gain1 : Gain  Gain=controller.lamxT2
  Gain3 : Gain  Gain=controller.lamTh2
  Scope : Scope  NumInputPorts=2
  Scope3 : Scope  NumInputPorts=2
  Scope5 : Scope  NumInputPorts=2
  Sum : Sum  Inputs=|+-
  Sum1 : Sum  Inputs=++|
  Sum2 : Sum  Inputs=|+-
  Sum3 : Sum  Inputs=++|
  Sum6 : Sum  Inputs=|+-
  Sum7 : Sum  Inputs=++|
  theta1VelocityDesired : Sin  Amplitude=pathPlanner.theta1A  Bias=pathPlanner.theta1B  Frequency=pathPlanner.theta1f  SampleTime=0
  theta2VelocityDesired : Sin  Amplitude=pathPlanner.theta2A  Bias=pathPlanner.theta2B  Frequency=pathPlanner.theta2f  SampleTime=0
  xt2VelocityDesired : Sin  Amplitude=pathPlanner.xt2A  Bias=pathPlanner.xt2B  Frequency=pathPlanner.xt2f  SampleTime=0
  jointVelocitiesRequired : Outport
  wires:
  Bus Creator/1 -> jointVelocitiesRequired/1  "jointVelocitiesRequired"
  [theta1VelReq] -> Bus Creator/1  "theta1VelocityRequired"
  [theta2VelReq] -> Bus Creator/2  "theta2VelocityRequired"
  [xt2VelReq] -> Bus Creator/3  "xt2VelocityRequired"
  jointVariablesFiltered/1 -> Bus Selector/1  "jointVariablesFiltered"
  Bus Selector/1 -> [theta1Filt]  "<theta1Filtered>"
  Bus Selector/2 -> [theta2Filt]  "<theta2Filtered>"
  Bus Selector/3 -> [xt2Filt]  "<xt2Filtered>"
  Discrete-Time Integrator/1 -> [theta1Des], Sum/1  "theta1Desired"
  [theta1Filt] -> Sum/2  "theta1Filtered"
  Sum/1 -> Gain/1  "theta1Error"
  Gain/1 -> Sum1/2
  Sum1/1 -> [theta1VelReq]  "theta1VelocityRequired"
  theta1VelocityDesired/1 -> Sum1/1, Discrete-Time Integrator/1  "theta1VelocityDesired"
  theta2VelocityDesired/1 -> Sum7/1, Discrete-Time Integrator3/1  "theta2VelocityDesired"
  Sum7/1 -> [theta2VelReq]  "theta2VelocityRequired"
  Gain3/1 -> Sum7/2
  Sum6/1 -> Gain3/1  "theta2Error"
  Discrete-Time Integrator3/1 -> [theta2Des], Sum6/1  "theta2Desired"
  Discrete-Time Integrator1/1 -> [xt2Des], Sum2/1  "xt2Desired"
  [xt2Filt] -> Sum2/2  "xt2Filtered"
  Sum2/1 -> Gain1/1  "xt2Error"
  Gain1/1 -> Sum3/2
  xt2VelocityDesired/1 -> Sum3/1, Discrete-Time Integrator1/1  "xt2VelocityDesired"
  [theta1Filt] -> Scope/2  "theta1Filt"
  [theta1Des] -> Scope/1  "theta1Desired"
  [theta2Des] -> Scope3/1  "theta2Desired"
  [theta2Filt] -> Scope3/2  "theta2Filt"
  [xt2Filt] -> Scope5/2  "xt2Filt"
  [xt2Des] -> Scope5/1  "xt2Desired"
  [theta2Filt] -> Sum6/2  "theta2Filtered"
  Sum3/1 -> [xt2VelReq]  "xt2VelocityRequired"

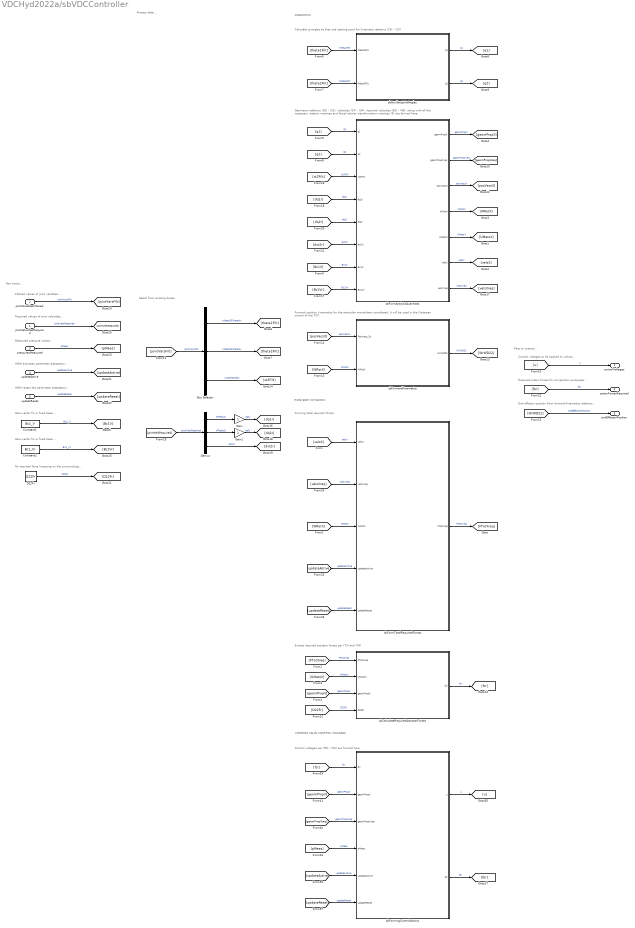
== system VDCHyd2022a/sbVDCController ==
  note: KINEMATICS
  note: Control voltages per (90) - (93) are formed here.
  note: Extract required actuator forces per (73) and (76).
  note: Forming total required forces.
  note: Forward position kinematics for the particular manipulator considered. It will be used in the Cartesian control of the TCP.
  note: Geometric relations (18) - (23), velocities (24) - (34), required velocities (38) - (48), along with all the necessary rotation
      | matrices and force/velocity transformation matrices (5) are formed here.
  note: Calculate qj angles as they are starting point for kinematic relations (18) - (23).
  note: End effector position from forward-kinematics relations...
  note: Control voltages to be applied to valves...
  note: Required piston forces for comparison puroposes...
  note: Select from existing buses...
  note: No required force imposing on the surroundings...
  note: Zero-vector for a fixed base....
  note: Zero-vector for a fixed base....
  note: HIGH resets the parameter adaptation...
  note: Measured pressure values...
  note: HIGH activates parameter adaptation...
  note: Required values of joint velocities...
  note: Filtered values of joint variables...
  note: Process data...
  note: Get inputs...
  note: Pass to outputs...
  note: RIGID BODY DYNAMICS
  note: FORMING VALVE CONTROL VOLTAGES
  jointVelocitiesRequired : Inport
  jointVariablesFiltered : Inport  Port=2
  pressuresMeasured : Inport  Port=3
  updateActive : Inport  Port=4
  updateReset : Inport  Port=5
  Bus Selector : BusSelector  OutputSignals=theta1Filtered,theta2Filtered,xt2Filtered
  Constant1 : Constant  Value=Bc1_V
  Constant2 : Constant  Value=Bc1_Vr
  D22Fr : Constant  Value=D22Fr
  Demux : Demux  Outputs=3
  Gain : Gain
  Gain1 : Gain
  sbAuxiliaryJointAngles : Subsystem
      mask Display: image('$imagefile'); % Use "Edit Image" on toolstrip to change.
  sbCalculateRequiredActuatorForces : Subsystem
  sbFormAnalyticQuantities : Subsystem
      mask Display: image('$imagefile'); % Use "Edit Image" on toolstrip to change.
  sbFormTotalRequiredForces : Subsystem
      mask Display: image('$imagefile'); % Use "Edit Image" on toolstrip to change.
  sbFormingControlActions : Subsystem
  sbForwardKinematics : Subsystem
      mask Display: image('$imagefile'); % Use "Edit Image" on toolstrip to change.
  controlVoltages : Outport
  pistonForcesRequired : Outport  Port=2
  endEffectorPosition : Outport  Port=3
  wires:
  updateActive/1 -> [updateActive]  "updateActive"
  [pMeas] -> sbFormingControlActions/4(pMeas)  "pMeas"
  [updateReset] -> sbFormingControlActions/6(updateReset)  "updateReset"
  sbFormingControlActions/1(u) -> [u]  "u"
  [updateActive] -> sbFormTotalRequiredForces/4(updateActive)  "updateActive"
  Bus Selector/3 -> [xt2Filt]  "<xt2Filtered>"
  [updateActive] -> sbFormingControlActions/5(updateActive)  "updateActive"
  Bus Selector/2 -> [theta2Filt]  "<theta2Filtered>"
  updateReset/1 -> [updateReset]  "updateReset"
  sbFormAnalyticQuantities/2(geomPropXreq) -> [geomPropXreq]  "geomPropXreq"
  [u] -> controlVoltages/1  "u"
  [Bc1V] -> sbFormAnalyticQuantities/7(Bc1V)  "Bc1V"
  [WrWD22] -> endEffectorPosition/1  "endEffectorPosition"
  [D22Fr] -> sbCalculateRequiredActuatorForces/4(D22Fr)  "D22Fr"
  sbFormAnalyticQuantities/3(posVecsX) -> [posVecsX]  "posVecsX"
  sbForwardKinematics/1(WrWD22) -> [WrWD22]  "WrWD22"
  sbAuxiliaryJointAngles/1(q1) -> [q1]  "q1"
  [posVecsX] -> sbForwardKinematics/1(PosVecs_Sx)  "posVecsX"
  [xt2Filt] -> sbFormAnalyticQuantities/3(xt2Filt)  "xt2Filt"
  [dq2r] -> sbFormAnalyticQuantities/5(dq2r)  "dq2r"
  [jointVelsRequired] -> Demux/1  "jointVelsRequired"
  [jointVarsFilt] -> Bus Selector/1  "jointVarsFilt"
  [dxt2r] -> sbFormAnalyticQuantities/6(dxt2r)  "dxt2r"
  [WRotX] -> sbFormTotalRequiredForces/3(WRotX)  "WRotX"
  Demux/3 -> [dxt2r]  "dxt2r"
  sbFormAnalyticQuantities/7(velsXreq) -> [velsXreq]  "velsXreq"
  [Bc1Vr] -> sbFormAnalyticQuantities/8(Bc1Vr)  "Bc1Vr"
  Gain1/1 -> [dq2r]  "dq2r"
  sbFormTotalRequiredForces/1(FTotXreq) -> [FTotXreq]  "FTotXreq"
  [velsX] -> sbFormTotalRequiredForces/1(velsX)  "velsX"
  [fcr] -> sbFormingControlActions/1(fcr)  "fcr"
  [FTotXreq] -> sbCalculateRequiredActuatorForces/1(FTotXreq)  "FTotXreq"
  [geomPropX] -> sbCalculateRequiredActuatorForces/3(geomPropX)  "geomPropX"
  [velsXreq] -> sbFormTotalRequiredForces/2(velsXreq)  "velsXreq"
  Constant2/1 -> [Bc1Vr]  "Bc1_Vr"
  Constant1/1 -> [Bc1V]  "Bc1_V"
  [updateReset] -> sbFormTotalRequiredForces/5(updateReset)  "updateReset"
  sbFormAnalyticQuantities/5(UMatsX) -> [UMatsX]  "UMatsX"
  pressuresMeasured/1 -> [pMeas]  "pMeas"
  sbFormAnalyticQuantities/1(geomPropX) -> [geomPropX]  "geomPropX"
  [theta2Filt] -> sbAuxiliaryJointAngles/2(theta2Filt)  "theta2Filt"
  [theta1Filt] -> sbAuxiliaryJointAngles/1(theta1Filt)  "theta1Filt"
  sbFormAnalyticQuantities/4(WRotX) -> [WRotX]  "WRotX"
  [dq1r] -> sbFormAnalyticQuantities/4(dq1r)  "dq1r"
  D22Fr/1 -> [D22Fr]  "D22Fr"
  [WRotX] -> sbForwardKinematics/2(WRotX)  "WRotX"
  [UMatsX] -> sbCalculateRequiredActuatorForces/2(UMatsX)  "UMatsX"
  [q2] -> sbFormAnalyticQuantities/2(q2)  "q2"
  [q1] -> sbFormAnalyticQuantities/1(q1)  "q1"
  sbAuxiliaryJointAngles/2(q2) -> [q2]  "q2"
  sbFormAnalyticQuantities/6(velsX) -> [velsX]  "velsX"
  Gain/1 -> [dq1r]  "dq1r"
  Bus Selector/1 -> [theta1Filt]  "<theta1Filtered>"
  jointVariablesFiltered/1 -> [jointVarsFilt]  "jointVarsFilt"
  jointVelocitiesRequired/1 -> [jointVelsRequired]  "jointVelsRequired"
  sbCalculateRequiredActuatorForces/1(fcr) -> [fcr]  "fcr"
  Demux/1 -> Gain/1  "dTheta1r"
  Demux/2 -> Gain1/1  "dTheta2r"
  sbFormingControlActions/2(fpr) -> [fpr]  "fpr"
  [fpr] -> pistonForcesRequired/1  "fpr"
  [geomPropX] -> sbFormingControlActions/2(geomPropX)  "geomPropX"
  [geomPropXreq] -> sbFormingControlActions/3(geomPropXreq)  "geomPropXreq"

== system VDCHyd2022a/sbFilterJointVariables/sbTheta1LowPassFilter ==
  theta1Measured : Inport
  Delay : Delay  InitialConditionSource=Input port  SampleTime=filtEnc.dT
      settings: InputPortMap=u0,p4
  Delay1 : Delay  DelayLength=1  InitialConditionSource=Input port  SampleTime=filtEnc.dT
      settings: InputPortMap=u0,p4
  Delay2 : Delay  DelayLength=0  InitialConditionSource=Input port  SampleTime=filtEnc.dT
      settings: InputPortMap=u0,p4
  Delay3 : Delay  InitialConditionSource=Input port  SampleTime=filtEnc.dT
      settings: InputPortMap=u0,p4
  Delay4 : Delay  DelayLength=1  InitialConditionSource=Input port  SampleTime=filtEnc.dT
      settings: InputPortMap=u0,p4
  Gain : Gain  Gain=filtEnc.a0
  Gain1 : Gain  Gain=filtEnc.b1
  Gain2 : Gain  Gain=filtEnc.b2
  Gain3 : Gain  Gain=filtEnc.b0
  Gain4 : Gain  Gain=filtEnc.a1
  Sum : Sum  Inputs=|--+++
  theta1Filtered : Outport
  wires:
  Gain3/1 -> Sum/5
  Sum/1 -> theta1Filtered/1, Delay4/1, Delay/1  "theta1Filtered"
  Delay2/1 -> Gain2/1
  Delay/1 -> Gain/1
  Delay1/1 -> Gain1/1
  Gain4/1 -> Sum/1
  Delay4/1 -> Gain4/1
  Gain2/1 -> Sum/3
  theta1Measured/1 -> Delay4/2, Delay/2, Delay2/1, Delay2/2, Delay1/1, Delay3/2, Delay3/1, Delay1/2  "theta1Measured"
  Delay3/1 -> Gain3/1
  Gain/1 -> Sum/2
  Gain1/1 -> Sum/4

== system VDCHyd2022a/sbFilterJointVariables/sbTheta2LowPassFilter ==
  theta2Measured : Inport
  Delay : Delay  InitialConditionSource=Input port  SampleTime=filtEnc.dT
      settings: InputPortMap=u0,p4
  Delay1 : Delay  DelayLength=1  InitialConditionSource=Input port  SampleTime=filtEnc.dT
      settings: InputPortMap=u0,p4
  Delay2 : Delay  DelayLength=0  InitialConditionSource=Input port  SampleTime=filtEnc.dT
      settings: InputPortMap=u0,p4
  Delay3 : Delay  InitialConditionSource=Input port  SampleTime=filtEnc.dT
      settings: InputPortMap=u0,p4
  Delay4 : Delay  DelayLength=1  InitialConditionSource=Input port  SampleTime=filtEnc.dT
      settings: InputPortMap=u0,p4
  Gain : Gain  Gain=filtEnc.a0
  Gain1 : Gain  Gain=filtEnc.b1
  Gain2 : Gain  Gain=filtEnc.b2
  Gain3 : Gain  Gain=filtEnc.b0
  Gain4 : Gain  Gain=filtEnc.a1
  Sum : Sum  Inputs=|--+++
  theta2Filtered : Outport
  wires:
  Gain3/1 -> Sum/5
  Gain2/1 -> Sum/3
  Delay4/1 -> Gain4/1
  Delay/1 -> Gain/1
  Delay1/1 -> Gain1/1
  Delay2/1 -> Gain2/1
  Gain4/1 -> Sum/1
  Sum/1 -> theta2Filtered/1, Delay4/1, Delay/1  "theta2Filtered"
  Gain1/1 -> Sum/4
  Gain/1 -> Sum/2
  Delay3/1 -> Gain3/1
  theta2Measured/1 -> Delay4/2, Delay/2, Delay2/1, Delay2/2, Delay1/1, Delay3/2, Delay3/1, Delay1/2  "theta2Measured"

== system VDCHyd2022a/sbFilterJointVariables/sbxt2LowPassFilter ==
  xt2Measured : Inport
  Delay : Delay  InitialConditionSource=Input port  SampleTime=filtEnc.dT
      settings: InputPortMap=u0,p4
  Delay1 : Delay  DelayLength=1  InitialConditionSource=Input port  SampleTime=filtEnc.dT
      settings: InputPortMap=u0,p4
  Delay2 : Delay  DelayLength=0  InitialConditionSource=Input port  SampleTime=filtEnc.dT
      settings: InputPortMap=u0,p4
  Delay3 : Delay  InitialConditionSource=Input port  SampleTime=filtEnc.dT
      settings: InputPortMap=u0,p4
  Delay4 : Delay  DelayLength=1  InitialConditionSource=Input port  SampleTime=filtEnc.dT
      settings: InputPortMap=u0,p4
  Gain : Gain  Gain=filtEnc.a0
  Gain1 : Gain  Gain=filtEnc.b1
  Gain2 : Gain  Gain=filtEnc.b2
  Gain3 : Gain  Gain=filtEnc.b0
  Gain4 : Gain  Gain=filtEnc.a1
  Sum : Sum  Inputs=|--+++
  xt2Filtered : Outport
  wires:
  Gain/1 -> Sum/2
  xt2Measured/1 -> Delay2/1, Delay2/2, Delay1/1, Delay3/2, Delay3/1, Delay1/2, Delay4/2, Delay/2  "xt2Measured"
  Delay2/1 -> Gain2/1
  Sum/1 -> xt2Filtered/1, Delay4/1, Delay/1  "xt2Filtered"
  Gain4/1 -> Sum/1
  Gain2/1 -> Sum/3
  Gain3/1 -> Sum/5
  Delay1/1 -> Gain1/1
  Delay3/1 -> Gain3/1
  Delay/1 -> Gain/1
  Delay4/1 -> Gain4/1
  Gain1/1 -> Sum/4
